simulink model "launch"  (R2025a)
settings: Solver=FixedStepAuto  StartTime=0.0  StopTime=0.7  FixedStep=1e-5  RelTol=1e-3
values from neighbouring files (symbols this model uses):
  CD = 0.3    [launch_data.sldd]
  CL = 1.2    [launch_data.sldd]
  density = 1.0    [launch_data.sldd]
  F = 600.0    [launch_data.sldd]
  fric = 0.1    [launch_data.sldd]
  g = 9.80665    [launch_data.sldd]
  m = 20.0    [launch_data.sldd]
  miu2 = 0.882    [launch_data.sldd]
  S1 = 0.23    [launch_data.sldd]
  S2 = 1.3    [launch_data.sldd]
  theta = 0.1047    [launch_data.sldd]
settings Model: DataDictionary=launch_data.sldd  Creator=MangoJuice  LastModifiedBy=MangoJuice

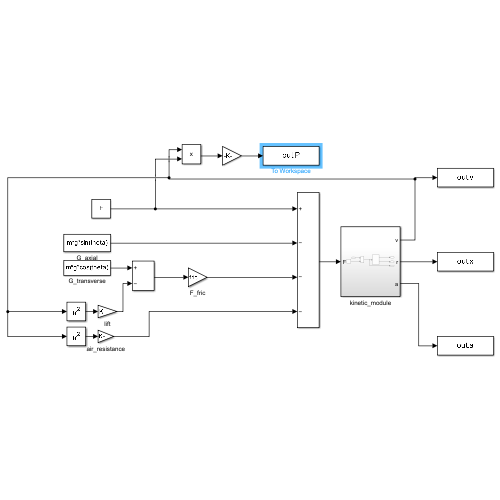
[thumbnail: Simulink's stored preview of the top-level diagram]
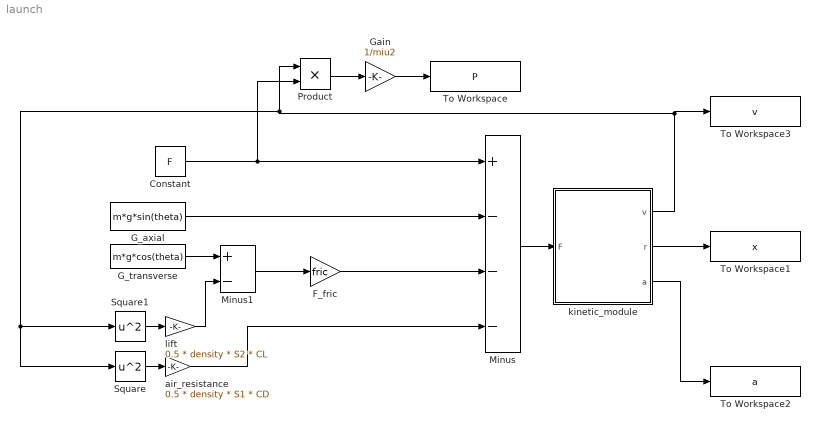
== system launch ==
  Constant : Constant  Value=F
  F_fric : Gain  Gain=fric
  G_axial : Constant  Value=m*g*sin(theta)
  G_transverse : Constant  Value=m*g*cos(theta)
  Gain : Gain  Gain=1/miu2
  Minus : Sum  Inputs=+---
  Minus1 : Sum  Inputs=+-
  Product : Product
  Square : Math  Operator=square
  Square1 : Math  Operator=square
  To Workspace : ToWorkspace  VariableName=P  SaveFormat=Timeseries  SampleTime=-1
  To Workspace1 : ToWorkspace  VariableName=x  SaveFormat=Timeseries  SampleTime=-1
  To Workspace2 : ToWorkspace  VariableName=a  SaveFormat=Timeseries  SampleTime=-1
  To Workspace3 : ToWorkspace  VariableName=v  SaveFormat=Timeseries  SampleTime=-1
  air_resistance : Gain  Gain=0.5 * density * S1 * CD
  kinetic_module : Subsystem
  lift : Gain  Gain=0.5 * density * S2 * CL
  wires:
  kinetic_module/1(v) -> To Workspace3/1, Product/1, Square/1, Square1/1
  Square/1 -> air_resistance/1
  Square1/1 -> lift/1
  Minus/1 -> kinetic_module/1(F)
  G_transverse/1 -> Minus1/1
  lift/1 -> Minus1/2
  Minus1/1 -> F_fric/1
  Constant/1 -> Product/2, Minus/1
  G_axial/1 -> Minus/2
  F_fric/1 -> Minus/3
  air_resistance/1 -> Minus/4
  kinetic_module/2(r) -> To Workspace1/1
  kinetic_module/3(a) -> To Workspace2/1
  Product/1 -> Gain/1
  Gain/1 -> To Workspace/1

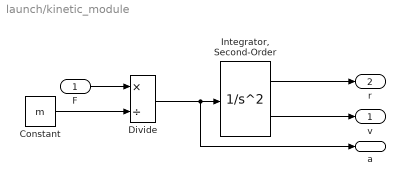
== system launch/kinetic_module ==
  F : Inport
  Constant : Constant  Value=m
  Divide : Product  Inputs=*/
  "Integrator, Second-Order" : SecondOrderIntegrator
  v : Outport
  r : Outport  Port=2
  a : Outport  Port=3
  wires:
  F/1 -> Divide/1
  Constant/1 -> Divide/2
  Divide/1 -> "Integrator, Second-Order"/1, a/1
  "Integrator, Second-Order"/2 -> v/1
  "Integrator, Second-Order"/1 -> r/1
